simulink model "AGC30Model_ex1_11"  (R2021a)
settings: Solver=ode4  StartTime=stime  StopTime=etime  FixedStep=dtload  RelTol=1e-3
values from neighbouring files (symbols this model uses):
  AL_A = 0.3    [init_lfc_model.m]
  AL_B = 0.3    [init_lfc_model.m]
  DELTA_CC = Delta_cc_ty(TY_CC)    [load_thermal_constants.m]
  DELTA_ST = Delta_st_ty(TY_ST)    [load_thermal_constants.m]
  dtload = 0.1    [initset_dataload.m]
  F0 = 60    [init_inertia_model.m]    (also in initset_inertia.m)
  FFCS0_CC = (WF0_CC-WF_MIN_CC)./(1.0-WF_MIN_CC)    [calc_thermal_init_values.m]    (also in init_thermals.m)
  FGT_CC = Fgt_cc_ty(TY_CC)    [load_thermal_constants.m]
  FX_FB_CC = Fx_fb_cc_ty(:,TY_CC)    [load_thermal_constants.m]
  FX_FB_ST = Fx_fb_st_ty(:,TY_ST)    [load_thermal_constants.m]
  FX_FB_WT = FX_FB_WT_ty(:,TY_WT)    [load_const_hydro_constants.m]
  FX_N_GN_VA = FX_N_GN_VA_ty(:,TY_VA)    [load_var_hydro_constants.m]
  FX_N_PM_VA = FX_N_PM_VA_ty(:,TY_VA)    [load_var_hydro_constants.m]
  FX_PTHD_ST = Fx_pthd_st_ty(:,TY_ST)    [load_thermal_constants.m]
  FX_T_PM_VA = FX_T_PM_VA_ty(:,TY_VA)    [load_var_hydro_constants.m]
  FX_TE1_CC = Fx_te1_cc_ty(:,TY_CC)    [load_thermal_constants.m]
  FX_TE2_CC = Fx_te2_cc_ty(:,TY_CC)    [load_thermal_constants.m]
  FX_Y_GN_VA = FX_Y_GN_VA_ty(:,TY_VA)    [load_var_hydro_constants.m]
  FX_Y_PM_VA = FX_Y_PM_VA_ty(:,TY_VA)    [load_var_hydro_constants.m]
  FY_FB_CC = Fy_fb_cc_ty(:,TY_CC)    [load_thermal_constants.m]
  FY_FB_ST = Fy_fb_st_ty(:,TY_ST)    [load_thermal_constants.m]
  FY_FB_WT = FY_FB_WT_ty(:,TY_WT)    [load_const_hydro_constants.m]
  FY_N_GN_VA = FY_N_GN_VA_ty(:,TY_VA)    [load_var_hydro_constants.m]
  FY_N_PM_VA = FY_N_PM_VA_ty(:,TY_VA)    [load_var_hydro_constants.m]
  FY_PTHD_ST = Fy_pthd_st_ty(:,TY_ST)    [load_thermal_constants.m]
  FY_T_PM_VA = FY_T_PM_VA_ty(:,TY_VA)    [load_var_hydro_constants.m]
  FY_TE1_CC = Fy_te1_cc_ty(:,TY_CC)    [load_thermal_constants.m]
  FY_TE2_CC = Fy_te2_cc_ty(:,TY_CC)    [load_thermal_constants.m]
  FY_Y_GN_VA = FY_Y_GN_VA_ty(:,TY_VA)    [load_var_hydro_constants.m]
  FY_Y_PM_VA = FY_Y_PM_VA_ty(:,TY_VA)    [load_var_hydro_constants.m]
  G_cost = [Cost(:,3) ... (first row only)    [initset_dataload.m]
  G_down_limit = max(G_down_limit, G_out_pre - G_speed*5)    [calc_edc_output.m]    (also in edc.m; initset_dataload.m = csvread('G_down_plan_limit.csv',0,1))
  G_G_ST = G_g_st_ty(TY_ST)    [load_thermal_constants.m]
  G_speed = u(220:249,1)    [calc_edc_output.m]    (also in edc.m; initset_dataload.m = G_speed(:,1))
  GF_CC = [1, 1, 1, 1, 1,            1, 1, 1, 1, 1]    [init_thermal_model.m]
  GF_ST = [1, 1, 1, 1, 1, 1, 1,            1, 1, 1, 1,            1, 1, 1, 1, 1, 1]    [init_thermal_model.m]
  GMW_CC = Gmw_cc_ty(TY_CC)    [load_thermal_constants.m]
  GMW_ST = Gmw_st_ty(TY_ST)    [load_thermal_constants.m]
  GMW_VA = GMW_VA_ty(TY_VA)    [load_var_hydro_constants.m]
  GMW_WT = GMW_WT_ty(TY_WT)    [load_const_hydro_constants.m]
  HC_CC = Hc_cc_ty(TY_CC)    [load_thermal_constants.m]
  HT_CC = Ht_cc_ty(TY_CC)    [load_thermal_constants.m]
  IGV0_CC = WF0_CC    [calc_thermal_init_values.m]    (also in init_thermals.m)
  inertia_input = inertia_input'    [initset_dataload.m]
  K1_CONV_VA = K1_CONV_VA_ty(TY_VA)    [load_var_hydro_constants.m]
  K1_CONV_WT = K1_CONV_WT_ty(TY_WT)    [load_const_hydro_constants.m]
  K2_SERV_VA = K2_SERV_VA_ty(TY_VA)    [load_var_hydro_constants.m]
  K2_SERV_WT = K2_SERV_WT_ty(TY_WT)    [load_const_hydro_constants.m]
  K_A = 0.1    [init_lfc_model.m]
  K_B = 0.1    [init_lfc_model.m]
  K_G_ST = K_g_st_ty(TY_ST)    [load_thermal_constants.m]
  K_IGV_CC = K_igv_cc_ty(TY_CC)    [load_thermal_constants.m]
  K_L = 2.0    (= 2)    [init_inertia_model.m]    (also in initset_inertia.m)
  K_MW_GV_VA = K_MW_GV_VA_ty(TY_VA)    [load_var_hydro_constants.m]
  K_PREF_ST = K_pref_st_ty(TY_ST)    [load_thermal_constants.m]
  K_SD_VA = K_SD_VA_ty(TY_VA)    [load_var_hydro_constants.m]
  K_SD_WT = K_SD_WT_ty(TY_WT)    [load_const_hydro_constants.m]
  K_SEQ_WT = K_SEQ_WT_ty(TY_WT)    [load_const_hydro_constants.m]
  K_TE_CC = K_te_cc_ty(TY_CC)    [load_thermal_constants.m]
  KD_PID_VA = KD_PID_VA_ty(TY_VA)    [load_var_hydro_constants.m]
  KD_PID_WT = KD_PID_WT_ty(TY_WT)    [load_const_hydro_constants.m]
  KD_SG_GN_VA = KD_SG_GN_VA_ty(TY_VA)    [load_var_hydro_constants.m]
  KD_SG_PM_VA = KD_SG_PM_VA_ty(TY_VA)    [load_var_hydro_constants.m]
  KGT_CC = FGT_CC./((TFR_CC-TER_CC)-(TDR_CC-TIR_CC))    [calc_thermal_init_values.m]    (also in init_thermals.m)
  KI_PID_VA = KI_PID_VA_ty(TY_VA)    [load_var_hydro_constants.m]
  KI_PID_WT = KI_PID_WT_ty(TY_WT)    [load_const_hydro_constants.m]
  KI_SG_GN_VA = KI_SG_GN_VA_ty(TY_VA)    [load_var_hydro_constants.m]
  KI_SG_PM_VA = KI_SG_PM_VA_ty(TY_VA)    [load_var_hydro_constants.m]
  KP_A = 1.0    (= 1)    [init_lfc_model.m]
  KP_B = 1.0    (= 1)    [init_lfc_model.m]
  KP_PID_VA = KP_PID_VA_ty(TY_VA)    [load_var_hydro_constants.m]
  KP_PID_WT = KP_PID_WT_ty(TY_WT)    [load_const_hydro_constants.m]
  KP_SG_GN_VA = KP_SG_GN_VA_ty(TY_VA)    [load_var_hydro_constants.m]
  KP_SG_PM_VA = KP_SG_PM_VA_ty(TY_VA)    [load_var_hydro_constants.m]
  KST_CC = (1.0-FGT_CC)./TER_CC    [calc_thermal_init_values.m]    (also in init_thermals.m)
  L_FUEL_CC = L_fuel_cc_ty(TY_CC)    [load_thermal_constants.m]
  L_G_ST = L_g_st_ty(TY_ST)    [load_thermal_constants.m]
  L_IGV_CC = L_igv_cc_ty(TY_CC)    [load_thermal_constants.m]
  L_LL_ST = L_ll_st_ty(TY_ST)    [load_thermal_constants.m]
  L_MWD_CC = L_mwd_cc_ty(TY_CC)    [load_thermal_constants.m]
  L_MWD_GN_VA = L_MWD_GN_VA_ty(TY_VA)    [load_var_hydro_constants.m]
  L_MWD_PM_VA = L_MWD_PM_VA_ty(TY_VA)    [load_var_hydro_constants.m]
  L_MWD_ST = L_mwd_st_ty(TY_ST)    [load_thermal_constants.m]
  L_MWD_WT = L_MWD_WT_ty(TY_WT)    [load_const_hydro_constants.m]
  L_PREF_CC = L_pref_cc_ty(TY_CC)    [load_thermal_constants.m]
  L_PREF_ST = L_pref_st_ty(TY_ST)    [load_thermal_constants.m]
  LFC_cycle = 5.0    (= 5)    [init_lfc_model.m]
  load_input = load_input(:,stime+1:etime+1)    [initset_dataload.m]
  M_VA = M_VA_ty(TY_VA)    [load_var_hydro_constants.m]
  MVABase = 1000    [init_inertia_model.m]    (also in initset_inertia.m)
  MW0_ST = zeros(1,17)    [calc_thermal_init_values.m]    (also in init_thermals.m)
  MW0_WT = zeros(1,2)    [calc_const_hydro_init_values.m]    (also in init_conhydros.m)
  P_G_CONV_WT = P_G_CONV_WT_ty(TY_WT)    [load_const_hydro_constants.m]
  PG_INIT_CC = PMWD_SCHEDULE(1,19:28)'    [calc_thermal_init_values.m]    (also in init_thermals.m)
  PLM_CC = Plm_cc_ty(TY_CC)    [load_thermal_constants.m]
  PLM_ST = Plm_st_ty(TY_ST)    [load_thermal_constants.m]
  PMAX_B = 360.0    (= 360)    [init_lfc_model.m]
  PMIN_B = -360.0    (= -360)    [init_lfc_model.m]
  PMST0_CC = zeros(1, 10)    [calc_thermal_init_values.m]    (also in init_thermals.m)
  PMWD_EDC0 = zeros(1,30)    [init_edc_model.m]    (also in initset_edc.m)
  PMWD_SCHEDULE = u(3:32,1)    [calc_edc_output.m]    (also in edc.m; init_edc_model.m = g_out_input'; initset_edc.m = g_out_input')
  PRC_CC = Prc_cc_ty(TY_CC)    [load_thermal_constants.m]
  PRT_CC = PRC_CC.*(1-EP_CC)    [calc_thermal_init_values.m]    (also in init_thermals.m)
  PTH0_ST = zeros(1,17)    [calc_thermal_init_values.m]    (also in init_thermals.m)
  R_LL_ST = R_ll_st_ty(TY_ST)    [load_thermal_constants.m]
  R_MWD_CC = R_mwd_cc_ty(TY_CC)    [load_thermal_constants.m]
  R_MWD_ST = R_mwd_st_ty(TY_ST)    [load_thermal_constants.m]
  R_PREF_CC = R_pref_cc_ty(TY_CC)    [load_thermal_constants.m]
  RA_A = G_speed'    [init_lfc_model.m]
  RA_B = 96.0    (= 96)    [init_lfc_model.m]
  RATE_GN_VA = RATE_GN_VA_ty(TY_VA)    [load_var_hydro_constants.m]
  RATE_PM_VA = RATE_PM_VA_ty(TY_VA)    [load_var_hydro_constants.m]
  RC_CC = Rc_cc_ty(TY_CC)    [load_thermal_constants.m]
  RT_CC = Rt_cc_ty(TY_CC)    [load_thermal_constants.m]
  SW_T_ST = Sw_t_st_ty(TY_ST)    [load_thermal_constants.m]
  T1_B_ST = T1_b_st_ty(TY_ST)    [load_thermal_constants.m]
  T1_CONV_VA = T1_CONV_VA_ty(TY_VA)    [load_var_hydro_constants.m]
  T1_CONV_WT = T1_CONV_WT_ty(TY_WT)    [load_const_hydro_constants.m]
  T1_G_ST = T1_g_st_ty(TY_ST)    [load_thermal_constants.m]
  T2_B_ST = T2_b_st_ty(TY_ST)    [load_thermal_constants.m]
  ... (+53 more)
undefined symbols (not defined in the file or in its folder): DELTA_B, DiscIntNeverNeededParam, FX_FB_ST_OA, FX_PTHD_ST_OA, FY_FB_ST_OA, FY_PTHD_ST_OA, G_G_ST_OA, K_G_ST_OA, K_PREF_ST_OA, MW0_ST_OA, N_GN_INIT_VA, N_PM_INIT_VA, PLM_B, R_LL_ST_OA, T1_B_ST_OA, T1_G_ST_OA, T2_B_ST_OA, T2_G_ST_OA, T3_B_ST_OA, T4_G_ST_OA, T5_G_ST_OA, T_LL_ST_OA, T_PREF_ST_OA, Y_GN_INIT_VA, Y_PM_INIT_VA
libraries: simulink_extras x87, simulink x42, pid_lib x1
(part 1 of 5)
settings Model: SimulationMode=accelerator  Creator=h-amano  LastModifiedBy=PowerSystemLab
settings SolverCC: AlgebraicLoopSolver=LineSearch
settings DataIOCC: LimitDataPoints=on  SaveFormat=Array  ReturnWorkspaceOutputs=off
settings OptimizationCC: ExpressionDepthLimit=2147483647  LifeSpan=inf
settings DebuggingCC: AlgebraicLoopMsg=none  ArtificialAlgebraicLoopMsg=none  UnderspecifiedInitializationDetection=Classic  MergeDetectMultiDrivingBlocksExec=none  SolverPrmCheckMsg=warning  InheritedTsInSrcMsg=none  MultiTaskRateTransMsg=warning  FcnCallInpInsideContextMsg=warning  StateNameClashWarn=warning  SFUnexpectedBacktrackingDiag=warning  SFNoUnconditionalDefaultTransitionDiag=warning  SFExecutionAtInitializationDiag=none  SFMachineParentedDataDiag=warning  ArithmeticOperatorsInVariantConditions=warning
settings HardwareCC: ProdBitPerPointer=32  ProdBitPerSizeT=32  ProdBitPerPtrDiffT=32  ProdLargestAtomicFloat=None  ProdIntDivRoundTo=Undefined  ProdEndianess=Unspecified  ProdWordSize=32  ProdHWDeviceType=32-bit Generic
settings ModelReferenceCC: PropagateSignalLabelsOutOfModel=off
settings SFSimCC: SimUseLocalCustomCode=off  CustomCodeUndefinedFunction=UseInterfaceOnly
settings RTWCC: RTWUseLocalCustomCode=off
settings CodeAppCC: StateflowObjectComments=on
settings GRTTargetCC: TargetLangStandard=C89/C90 (ANSI)  CombineOutputUpdateFcns=off  GRTInterface=on
settings ConfigComp: CovMetricSettings=dw  CovSaveCumulativeToWorkspaceVar=on  CovSaveSingleToWorkspaceVar=on  CovExternalEMLEnable=off  CovSFcnEnable=off

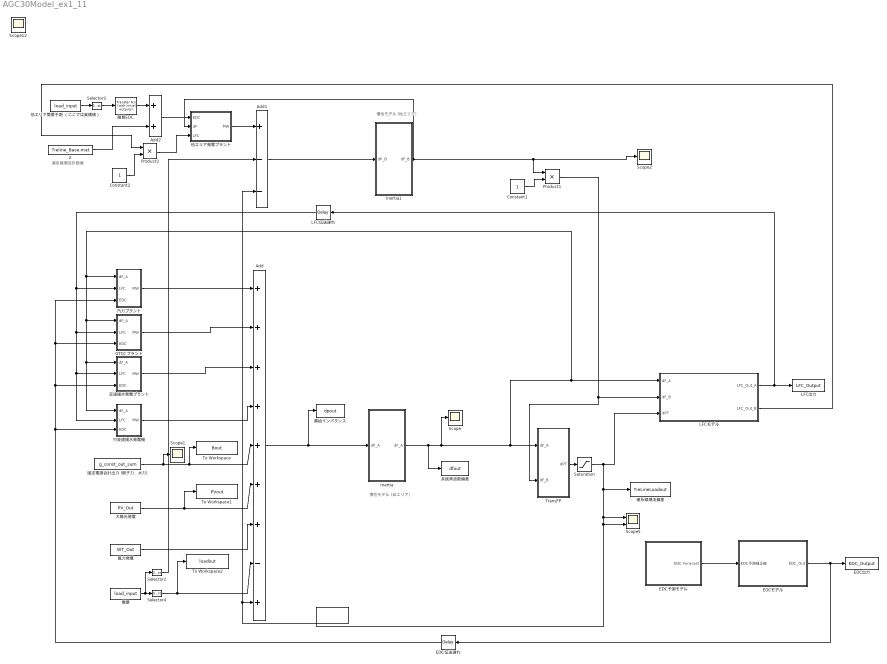
== system AGC30Model_ex1_11 ==
  note: 連系線潮流計画値
  note: 慣性モデル
      | (自エリア)
  note: 慣性モデル
      | (他エリア)
  "  2" : FromFile  FileName=Tieline_Base.mat  SampleTime=dtload
  Add : Sum  Inputs=+++++++-+
  Add1 : Sum  Inputs=+--
  Add2 : Sum
  Constant1 : Constant
  Constant2 : Constant
  EDCモデル : Subsystem
  EDC予測モデル : Subsystem
  EDC伝送遅れ : TransportDelay  DelayTime=3  InitialOutput=PMWD_EDC0
  EDC出力 : ToWorkspace  VariableName=EDC_Output  SampleTime=dtload
      settings: Decimation=10
  GTCCプラント : Subsystem
  Inertia : Subsystem
  Inertia1 : Subsystem
  LFCモデル : Subsystem
  LFC伝送遅れ : TransportDelay  DelayTime=3
  LFC出力 : ToWorkspace  VariableName=LFC_Output  SampleTime=dtload
      settings: Decimation=10
  Product1 : Product
  Product2 : Product
  Saturation : Saturate  UpperLimit=50  LowerLimit=-50
  Scope{,1..2,12} (4 alike) : Scope
  Scope5 : Scope  NumInputPorts=2
  Selector2 : Selector  InputPortWidth=2  IndexOptions=Index vector (dialog)  Indices=[2]  OutputSizes=1
  Selector3 : Selector  InputPortWidth=2  IndexOptions=Index vector (dialog)  Indices=[2]  OutputSizes=1
  Selector4 : Selector  InputPortWidth=2  IndexOptions=Index vector (dialog)  Indices=[1]  OutputSizes=1
  To Workspace : ToWorkspace  VariableName=Bout  SaveFormat=Timeseries  SampleTime=-1
      settings: Decimation=10
  To Workspace1 : ToWorkspace  VariableName=PVout  SaveFormat=Timeseries  SampleTime=-1
      settings: Decimation=10
  To Workspace2 : ToWorkspace  VariableName=loadout  SaveFormat=Timeseries  SampleTime=-1
      settings: Decimation=10
  TransFP : Subsystem
  他エリア発電プラント : Subsystem
  他エリア需要予測 （ここでは実績値） : FromFile  FileName=load_input  SampleTime=dtload
  可変速揚水発電機 : Subsystem
  固定電源合計出力 (原子力，水力) : FromFile  FileName=g_const_out_sum  SampleTime=dtload
  太陽光発電 : FromFile  FileName=PV_Out  SampleTime=dtload
  定速揚水発電プラント : Subsystem
  汽力プラント : Subsystem
  簡易EDC : simulink_extras/Additional Linear/Transfer Fcn (with initial outputs)  N=[1]  D="[200  1]"  Y0=load_input(3,1)  U0=load_input(3,1)
  系統周波数偏差 : ToWorkspace  VariableName=dfout  SampleTime=-1
      settings: Decimation=10  Save2DSignal=2-D array (concatenate along first dimension)
  連系線潮流偏差 : ToWorkspace  VariableName=TieLineLoadout  SampleTime=-1
      settings: Decimation=10  Save2DSignal=2-D array (concatenate along first dimension)
  需給インバランス : ToWorkspace  VariableName=dpout  SampleTime=-1
      settings: Decimation=10  Save2DSignal=2-D array (concatenate along first dimension)
  需要 : FromFile  FileName=load_input  SampleTime=dtload
  風力発電 : FromFile  FileName=WT_Out  SampleTime=dtload
  wires:
  固定電源合計出力 (原子力，水力)/1 -> Scope1/1, To Workspace/1, Add/5
  太陽光発電/1 -> To Workspace1/1, Add/6
  風力発電/1 -> Add/7
  LFCモデル/1(LFC_Out_A) -> LFC出力/1, LFC伝送遅れ/1
  可変速揚水発電機/1(MW) -> Add/4
  定速揚水発電プラント/1(MW) -> Add/3
  汽力プラント/1(MW) -> Add/1
  GTCCプラント/1(MW) -> Add/2
  Add/1 -> 需給インバランス/1, Inertia/1(dP_A)
  Inertia/1(dF_A) -> Scope/1, TransFP/1(dF_A), GTCCプラント/1(dF_A), 可変速揚水発電機/1(dF_A), 定速揚水発電プラント/1(dF_A), 汽力プラント/1(dF_A), LFCモデル/1(dF_A), 系統周波数偏差/1
  Selector4/1 -> To Workspace2/1, Add/8
  EDCモデル/1(EDC_Out) -> EDC出力/1, EDC伝送遅れ/1
  需要/1 -> Selector2/1, Selector4/1
  Selector2/1 -> Add1/2
  他エリア需要予測 （ここでは実績値）/1 -> Selector3/1
  "  2"/1 -> Add2/2
  Selector3/1 -> 簡易EDC/1
  簡易EDC/1 -> Add2/1
  EDC予測モデル/1(EDC Forecast) -> EDCモデル/1(EDC予測補正値)
  EDC伝送遅れ/1 -> 定速揚水発電プラント/3(EDC), GTCCプラント/3(EDC), 汽力プラント/3(EDC), 可変速揚水発電機/3(EDC)
  LFC伝送遅れ/1 -> 汽力プラント/2(LFC), GTCCプラント/2(LFC), 可変速揚水発電機/2(LFC), 定速揚水発電プラント/2(LFC)
  Add2/1 -> 他エリア発電プラント/1(EDC)
  LFCモデル/2(LFC_Out_B) -> Product2/1
  他エリア発電プラント/1(MW) -> Add1/1
  Constant2/1 -> Product2/2
  Product2/1 -> 他エリア発電プラント/3(LFC)
  Inertia1/1(dF_B) -> 他エリア発電プラント/2(dF), Scope2/1, Product1/1
  TransFP/1(dPT) -> Saturation/1
  Add1/1 -> Inertia1/1(dP_B)
  Constant1/1 -> Product1/2
  Product1/1 -> TransFP/2(dF_B), LFCモデル/2(dF_B)
  Saturation/1 -> 連系線潮流偏差/1, Scope5/1, Add/9, Add1/3, Scope5/2, LFCモデル/3(dPT)

== system AGC30Model_ex1_11/EDCモデル ==
  EDC予測補正値 : Inport
  Demux9 : Demux  Outputs=103
      settings: DisplayOption=none
  EDC計算のための入力データ : Subsystem
  Fcn : Fcn  Expr=u-2
  Mux : Mux  Inputs=30
  Mux1 : Mux  Inputs=30
  Mux2 : Mux  Inputs=30
  Mux3 : Mux  Inputs=7
  Mux5 : Mux
  Rate Limiter : RateLimiter  RisingSlewLimit=G_speed/60  FallingSlewLimit=-G_speed/60  SampleTimeMode=inherited  InitialCondition=PMWD_SCHEDULE(1,2:end)
  S-Function1 : S-Function  FunctionName=edc  SFunctionDeploymentMode=off  EnableBusSupport=off
  Switch : Switch  Criteria=u2 ~= 0  Threshold=2
  Switch1 : Switch  Criteria=u2 ~= 0  Threshold=2
  csv_output1 : ToWorkspace  VariableName=PMWD_EDC_O  SampleTime=300
  csv_output10 : ToWorkspace  VariableName=P0_O  SampleTime=300
  csv_output11 : ToWorkspace  VariableName=PMWD_EDC_O1  SampleTime=1
  csv_output2 : ToWorkspace  VariableName=EDC_haibun_O  SampleTime=300
  csv_output3 : ToWorkspace  VariableName=EDC_ERR_O  SampleTime=300
  csv_output4 : ToWorkspace  VariableName=P_OUT_O  SampleTime=300
  csv_output5 : ToWorkspace  VariableName=P_cost_O  SampleTime=300
  csv_output6 : ToWorkspace  VariableName=P_LOAD_A_AD_O  SampleTime=300
  csv_output7 : ToWorkspace  VariableName=P_plan_O  SampleTime=300
  csv_output8 : ToWorkspace  VariableName=G_MODE_O  SampleTime=300
  csv_output9 : ToWorkspace  VariableName=P_CONSTANT_O  SampleTime=300
  hatuden_keikaku : FromWorkspace  VariableName=PMWD_SCHEDULE  SampleTime=-1  ZeroCross=off  OutputAfterFinalValue=Holding final value
  hatudenki_mode : FromWorkspace  VariableName=G_MODE  SampleTime=-1  Interpolate=off  ZeroCross=off  OutputAfterFinalValue=Holding final value
  前回演算時の EDC出力 : UnitDelay  InitialCondition=PMWD_SCHEDULE(1,2:31)  SampleTime=-1  HasFrameUpgradeWarning=on
  発電機の出力変化速度 : Constant  Value=G_speed  SampleTime=-1
  EDC_Out : Outport  VectorParamsAs1DForOutWhenUnconnected=off
  wires:
  Mux/1 -> csv_output1/1, Switch/1
  Demux9/1 -> Mux/1
  Demux9/2 -> Mux/2
  Demux9/3 -> Mux/3
  Demux9/4 -> Mux/4
  Demux9/5 -> Mux/5
  Demux9/6 -> Mux/6
  Demux9/7 -> Mux/7
  Demux9/8 -> Mux/8
  Demux9/9 -> Mux/9
  Demux9/10 -> Mux/10
  Demux9/11 -> Mux/11
  Demux9/12 -> Mux/12
  Demux9/13 -> Mux/13
  Demux9/14 -> Mux/14
  Demux9/15 -> Mux/15
  Demux9/16 -> Mux/16
  Demux9/17 -> Mux/17
  Demux9/18 -> Mux/18
  Demux9/19 -> Mux/19
  Demux9/20 -> Mux/20
  Demux9/21 -> Mux/21
  Demux9/22 -> Mux/22
  Demux9/23 -> Mux/23
  Demux9/24 -> Mux/24
  Demux9/25 -> Mux/25
  Demux9/26 -> Mux/26
  Demux9/27 -> Mux/27
  Demux9/28 -> Mux/28
  Demux9/29 -> Mux/29
  Demux9/30 -> Mux/30
  S-Function1/1 -> Demux9/1
  EDC計算のための入力データ/1(EDC_data) -> Mux5/2
  Mux5/1 -> S-Function1/1
  EDC予測補正値/1 -> Mux5/1
  Mux2/1 -> csv_output8/1
  Demux9/102 -> Mux2/30
  Demux9/101 -> Mux2/29
  Demux9/100 -> Mux2/28
  Demux9/99 -> Mux2/27
  Demux9/98 -> Mux2/26
  Demux9/97 -> Mux2/25
  Demux9/96 -> Mux2/24
  Demux9/95 -> Mux2/23
  Demux9/94 -> Mux2/22
  Demux9/93 -> Mux2/21
  Demux9/92 -> Mux2/20
  Demux9/91 -> Mux2/19
  Demux9/90 -> Mux2/18
  Demux9/89 -> Mux2/17
  Demux9/88 -> Mux2/16
  Demux9/87 -> Mux2/15
  Demux9/85 -> Mux2/13
  Demux9/83 -> Mux2/11
  Demux9/82 -> Mux2/10
  Demux9/81 -> Mux2/9
  Demux9/80 -> Mux2/8
  Demux9/79 -> Mux2/7
  Demux9/78 -> Mux2/6
  Demux9/77 -> Mux2/5
  Demux9/76 -> Mux2/4
  Demux9/75 -> Mux2/3
  Demux9/74 -> Mux2/2
  Demux9/73 -> Mux2/1
  Demux9/72 -> csv_output7/1
  Demux9/71 -> csv_output6/1
  Mux1/1 -> csv_output5/1
  Demux9/41 -> Mux1/1
  Demux9/42 -> Mux1/2
  Demux9/43 -> Mux1/3
  Demux9/44 -> Mux1/4
  Demux9/45 -> Mux1/5
  Demux9/46 -> Mux1/6
  Demux9/47 -> Mux1/7
  Demux9/48 -> Mux1/8
  Demux9/49 -> Mux1/9
  Demux9/50 -> Mux1/10
  Demux9/51 -> Mux1/11
  Demux9/52 -> Mux1/12
  Demux9/53 -> Mux1/13
  Demux9/54 -> Mux1/14
  Demux9/55 -> Mux1/15
  Demux9/56 -> Mux1/16
  Demux9/57 -> Mux1/17
  Demux9/58 -> Mux1/18
  Demux9/59 -> Mux1/19
  Demux9/61 -> Mux1/21
  Demux9/62 -> Mux1/22
  Demux9/63 -> Mux1/23
  Demux9/64 -> Mux1/24
  Demux9/65 -> Mux1/25
  Demux9/66 -> Mux1/26
  Demux9/67 -> Mux1/27
  Demux9/68 -> Mux1/28
  Demux9/69 -> Mux1/29
  Demux9/70 -> Mux1/30
  Demux9/31 -> Mux3/1
  Demux9/32 -> Mux3/2
  Demux9/33 -> Mux3/3
  Demux9/34 -> Mux3/4
  Demux9/35 -> Mux3/5
  Demux9/36 -> Mux3/6
  Demux9/37 -> Mux3/7
  Mux3/1 -> csv_output9/1
  Demux9/60 -> Mux1/20
  Demux9/38 -> csv_output2/1
  Demux9/39 -> csv_output3/1
  Demux9/40 -> csv_output4/1
  Demux9/84 -> Mux2/12
  Demux9/86 -> Mux2/14
  Demux9/103 -> csv_output10/1
  hatudenki_mode/1 -> Fcn/1, Switch/2
  hatuden_keikaku/1 -> Switch1/3, Switch/3
  Switch/1 -> Switch1/1
  Fcn/1 -> Switch1/2
  前回演算時の EDC出力/1 -> Mux5/4
  発電機の出力変化速度/1 -> Mux5/3
  Switch1/1 -> Rate Limiter/1, 前回演算時の EDC出力/1, EDC_Out/1
  Rate Limiter/1 -> csv_output11/1

== system AGC30Model_ex1_11/EDC予測モデル ==
  EDC予測データ : ToWorkspace  VariableName=load_forcast_out  SampleTime=-1
      settings: Decimation=10  Save2DSignal=2-D array (concatenate along first dimension)
  Gain : Gain  Gain=1/200
  Integrator : Integrator  InitialConditionSource=external
  Mux : Mux  Inputs=2
  Mux1 : Mux  Inputs=3
  Scope : Scope
  Scope1 : Scope
  Selector2 : Selector  InputPortWidth=2  IndexOptions=Index vector (dialog)  Indices=[1]  OutputSizes=1
  Subtract : Sum  Inputs=+--
  Sum : Sum  Inputs=|+-
  Sum1 : Sum  Inputs=++|
  Sum2 : Sum  Inputs=|+-
  太陽光発電 : FromFile  FileName=PV_Out  SampleTime=dtload
  発電計画時の予測需要 : FromFile  FileName=load_forecast_input  SampleTime=dtload
  発電計画時の予測需要 （5分先） : FromFile  FileName=load_forecast_300s_input  SampleTime=dtload
  需要 : FromFile  FileName=load_input  SampleTime=dtload
  風力発電 : FromFile  FileName=WT_Out  SampleTime=dtload
  EDC Forecast : Outport  VectorParamsAs1DForOutWhenUnconnected=off
  wires:
  Gain/1 -> Integrator/1
  Sum1/1 -> Mux1/3, EDC Forecast/1
  需要/1 -> Selector2/1
  発電計画時の予測需要/1 -> Mux1/2, Sum/2, Mux/1
  Subtract/1 -> Mux1/1, Sum/1
  Mux/1 -> Scope/1
  Sum/1 -> Integrator/2, Sum2/1
  Sum2/1 -> Gain/1
  発電計画時の予測需要 （5分先）/1 -> Mux/2, Sum1/2
  Integrator/1 -> Sum1/1, Sum2/2
  Mux1/1 -> Scope1/1, EDC予測データ/1
  Selector2/1 -> Subtract/1
  太陽光発電/1 -> Subtract/2
  風力発電/1 -> Subtract/3

== system AGC30Model_ex1_11/GTCCプラント ==
  dF_A : Inport
  LFC : Inport  Port=2
  EDC : Inport  Port=3
  Add : Sum  Inputs=+
  EDC_Gtcc1 : Selector  InputPortWidth=AGCNum_E  IndexOptions=Index vector (dialog)  Indices=[18]  OutputSizes=1
  GTCC1 : Subsystem
  GTCCプラント出力 : ToWorkspace  VariableName=Combine_Output  SampleTime=-1
      settings: Decimation=10  Save2DSignal=2-D array (concatenate along first dimension)
  LFC_Gtcc1 : Selector  InputPortWidth=AGCNum_L  IndexOptions=Index vector (dialog)  Indices=[18]  OutputSizes=1
  Mux : Mux  Inputs=1
  To Workspace : ToWorkspace  VariableName=GTCC  SaveFormat=Timeseries  SampleTime=-1
      settings: Decimation=10
  MW : Outport  VectorParamsAs1DForOutWhenUnconnected=off
  wires:
  GTCC1/1(タービン出力(MW)) -> Add/1, To Workspace/1, Mux/1
  LFC/1 -> LFC_Gtcc1/1
  dF_A/1 -> GTCC1/3(周波数偏差(Hz))
  Mux/1 -> GTCCプラント出力/1
  LFC_Gtcc1/1 -> GTCC1/2(LFC指令値(MW))
  Add/1 -> MW/1
  EDC_Gtcc1/1 -> GTCC1/1(EDC指令値(MW))
  EDC/1 -> EDC_Gtcc1/1

== system AGC30Model_ex1_11/Inertia ==
  note: 系統容量
  note: 慣性定数
  note: 需給インバランス
      | (ΔP)
  dP_A : Inport  SampleTime=0.1
  "  1" : FromFile  FileName=inertia_input.mat  SampleTime=dtload
  "  2" : FromFile  FileName=load_input.mat  SampleTime=dtload
  Add2 : Sum  Inputs=+-
  Divide : Product  Inputs=/*
  Divide1 : Product  Inputs=/*
  Divide2 : Product  Inputs=**
  Selector1 : Selector  InputPortWidth=2  IndexOptions=Index vector (dialog)  Indices=[1]  OutputSizes=1
  Selector2 : Selector  InputPortWidth=2  IndexOptions=Index vector (dialog)  Indices=[1]  OutputSizes=1
  Transfer Fcn : TransferFcn  Denominator=[1 0]
  基準周波数 : Gain  Gain=F0
  系統容量基準値 : Constant  Value=MVABase
  負荷周波数特性係数 : Gain  Gain=K_L
  dF_A : Outport  VectorParamsAs1DForOutWhenUnconnected=off
  wires:
  負荷周波数特性係数/1 -> Divide2/2
  Divide/1 -> Divide1/2
  dP_A/1 -> Add2/1
  "  1"/1 -> Selector2/1
  Selector1/1 -> Divide2/1  "P_LOAD_A"
  基準周波数/1 -> dF_A/1  "d_F_A"
  Divide1/1 -> Transfer Fcn/1
  "  2"/1 -> Selector1/1
  Transfer Fcn/1 -> 負荷周波数特性係数/1, 基準周波数/1
  Add2/1 -> Divide/2
  Divide2/1 -> Add2/2
  系統容量基準値/1 -> Divide/1
  Selector2/1 -> Divide1/1  "M_0_A"

== system AGC30Model_ex1_11/Inertia1 ==
  note: 系統容量
  note: 慣性定数
  note: 需給インバランス
      | (ΔP)
  dP_B : Inport  SampleTime=0.1
  "  1" : FromFile  FileName=inertia_input.mat  SampleTime=dtload
  "  2" : FromFile  FileName=load_input.mat  SampleTime=dtload
  Add1 : Sum  Inputs=+-
  Divide : Product  Inputs=/*
  Divide1 : Product  Inputs=/*
  Divide2 : Product  Inputs=**
  Selector1 : Selector  InputPortWidth=2  IndexOptions=Index vector (dialog)  Indices=[2]  OutputSizes=1
  Selector2 : Selector  InputPortWidth=2  IndexOptions=Index vector (dialog)  Indices=[2]  OutputSizes=1
  Transfer Fcn : TransferFcn  Denominator=[1 0]
  基準周波数 : Gain  Gain=F0
  系統容量基準値 : Constant  Value=MVABase
  負荷周波数特性係数 : Gain  Gain=K_L
  dF_B : Outport  VectorParamsAs1DForOutWhenUnconnected=off
  wires:
  Transfer Fcn/1 -> 基準周波数/1, 負荷周波数特性係数/1
  "  2"/1 -> Selector1/1
  Divide1/1 -> Transfer Fcn/1
  基準周波数/1 -> dF_B/1  "d_F_B"
  "  1"/1 -> Selector2/1
  dP_B/1 -> Add1/1
  Selector2/1 -> Divide1/1  "M_0_A"
  系統容量基準値/1 -> Divide/1
  負荷周波数特性係数/1 -> Divide2/2
  Selector1/1 -> Divide2/1  "P_LOAD_A"
  Divide2/1 -> Add1/2
  Add1/1 -> Divide/2
  Divide/1 -> Divide1/2

== system AGC30Model_ex1_11/LFCモデル ==
  note: 連系線潮流計画値
  note: 系統容量
      | (需要データ)
  dF_A : Inport  SampleTime=dtload
  dF_B : Inport  Port=2  SampleTime=dtload
  dPT : Inport  Port=3  SampleTime=dtload
  "  1" : FromFile  FileName=load_input.mat  SampleTime=dtload
  "  2" : FromFile  FileName=Tieline_Base.mat  SampleTime=dtload
  Rate Transition : RateTransition  Deterministic=off  InitialCondition=load_input([2,3],1)  OutPortSampleTime=LFC_cycle
  Rate Transition1 : RateTransition  Deterministic=off  OutPortSampleTime=LFC_cycle
  Sum : Sum  Inputs=-+
  TBC/FFC 切替Switch : ManualSwitch
  TBC/FFC 切替Switch : ManualSwitch
  他エリア FFC方式 : Subsystem
  他エリア TBC方式 : Subsystem
  自エリア TBC方式 : Subsystem
  自エリアFFC方式 : Subsystem
  LFC_Out_A : Outport  VectorParamsAs1DForOutWhenUnconnected=off
  LFC_Out_B : Outport  Port=2  VectorParamsAs1DForOutWhenUnconnected=off
  wires:
  "  1"/1 -> Rate Transition/1
  Rate Transition/1 -> 自エリア TBC方式/1(系統容量(MW)), 自エリアFFC方式/1(系統容量(MW)), 他エリア TBC方式/1(系統容量(MW)), 他エリア FFC方式/1(系統容量(MW))
  自エリア TBC方式/1(LFC指令値(MW)) -> TBC/FFC 切替Switch/1
  自エリアFFC方式/1(LFC指令値(MW)) -> TBC/FFC 切替Switch/2
  TBC/FFC 切替Switch/1 -> LFC_Out_A/1
  dF_A/1 -> 自エリア TBC方式/2(周波数偏差(Hz)), 自エリアFFC方式/2(周波数偏差(Hz))
  他エリア TBC方式/1(LFC指令値(MW)) -> TBC/FFC 切替Switch/1
  他エリア FFC方式/1(LFC指令値(MW)) -> TBC/FFC 切替Switch/2
  TBC/FFC 切替Switch/1 -> LFC_Out_B/1
  dF_B/1 -> 他エリア TBC方式/2(周波数偏差(Hz)), 他エリア FFC方式/2(周波数偏差(Hz))
  "  2"/1 -> Sum/1
  dPT/1 -> Sum/2
  Sum/1 -> Rate Transition1/1
  Rate Transition1/1 -> 自エリア TBC方式/3(連系線潮流偏差(MW)), 他エリア TBC方式/3(連系線潮流偏差(Hz))

== system AGC30Model_ex1_11/TransFP ==
  dF_A : Inport
  dF_B : Inport  Port=2
  "  2" : FromFile  FileName=inertia_input.mat  SampleTime=dtload
  Add1 : Sum  Inputs=-+
  Add2 : Sum
  Constant1 : Constant  Value=2*pi/(F0*T_0^2)  SampleTime=dtload
  Divide : Product  Inputs=**
  Divide1 : Product  Inputs=//
  Divide2 : Product  Inputs=//
  Divide3 : Product  Inputs=/*
  F_0 : Gain  Gain=2*pi
  F_1 : Gain  Gain=2*pi
  Integrator : Integrator  InitialCondition=Tieline_Base(2,1)/(2*pi/(F0*T_0^2))*(1/(MVABase*inertia_input(2,1))+1/(MVABase*inertia_input(3,1)))
  Selector1 : Selector  InputPortWidth=2  IndexOptions=Index vector (dialog)  Indices=[1]  OutputSizes=1
  Selector3 : Selector  InputPortWidth=2  IndexOptions=Index vector (dialog)  Indices=[2]  OutputSizes=1
  系統容量基準値 : Constant  Value=MVABase
  dPT : Outport  SampleTime=dtload  VectorParamsAs1DForOutWhenUnconnected=off
  wires:
  Selector3/1 -> Divide2/1  "M_0_B"
  Selector1/1 -> Divide1/1  "M_0_A"
  Add1/1 -> Integrator/1
  "  2"/1 -> Selector3/1, Selector1/1
  dF_A/1 -> F_0/1
  dF_B/1 -> F_1/1
  Add2/1 -> Divide3/1
  Divide1/1 -> Add2/1
  Divide2/1 -> Add2/2
  Constant1/1 -> Divide3/2
  Divide3/1 -> Divide/1  "T_AB"
  F_0/1 -> Add1/1
  Divide/1 -> dPT/1  "DPT"
  F_1/1 -> Add1/2
  Integrator/1 -> Divide/2
  系統容量基準値/1 -> Divide2/2, Divide1/2

== system AGC30Model_ex1_11/他エリア発電プラント ==
  EDC : Inport
  dF : Inport  Port=2
  LFC : Inport  Port=3
  Scope : Scope  NumInputPorts=4
  他エリアモデル : Subsystem
  MW : Outport  VectorParamsAs1DForOutWhenUnconnected=off
  wires:
  他エリアモデル/1(タービン出力(MW)) -> Scope/4, MW/1
  EDC/1 -> Scope/3, 他エリアモデル/1(EDC指令値(MW))
  LFC/1 -> Scope/2, 他エリアモデル/2(LFC指令値(MW))
  dF/1 -> Scope/1, 他エリアモデル/3(周波数偏差(Hz))

== system AGC30Model_ex1_11/可変速揚水発電機 ==
  dF_A : Inport
  LFC : Inport  Port=2
  EDC : Inport  Port=3
  可変速揚水 : Subsystem
  可変速揚水機出力 : ToWorkspace  VariableName=C_Water_Output  SampleTime=-1
      settings: Decimation=10  Save2DSignal=2-D array (concatenate along first dimension)
  MW : Outport  VectorParamsAs1DForOutWhenUnconnected=off
  wires:
  EDC/1 -> 可変速揚水/1(EDC指令値 (MW))
  LFC/1 -> 可変速揚水/2(LFC指令値 (MW))
  dF_A/1 -> 可変速揚水/3(周波数偏差 (Hz))
  可変速揚水/1(発電機出力・揚水入力 (MW)) -> 可変速揚水機出力/1, MW/1

== system AGC30Model_ex1_11/定速揚水発電プラント ==
  dF_A : Inport
  LFC : Inport  Port=2
  EDC : Inport  Port=3
  Add : Sum
  EDC_Wt1 : Selector  InputPortWidth=AGCNum_E  IndexOptions=Index vector (dialog)  Indices=[28]  OutputSizes=1
  EDC_Wt2 : Selector  InputPortWidth=AGCNum_E  IndexOptions=Index vector (dialog)  Indices=[29]  OutputSizes=1
  LFC_Wt1 : Selector  InputPortWidth=AGCNum_L  IndexOptions=Index vector (dialog)  Indices=[28]  OutputSizes=1
  LFC_Wt2 : Selector  InputPortWidth=AGCNum_L  IndexOptions=Index vector (dialog)  Indices=[29]  OutputSizes=1
  Water1 : Subsystem
  Water2 : Subsystem
  定速揚水プラント出力1 : ToWorkspace  VariableName=Water_Output1  SampleTime=-1
      settings: Decimation=10  Save2DSignal=2-D array (concatenate along first dimension)
  定速揚水プラント出力2 : ToWorkspace  VariableName=Water_Output2  SampleTime=-1
      settings: Decimation=10  Save2DSignal=2-D array (concatenate along first dimension)
  MW : Outport  VectorParamsAs1DForOutWhenUnconnected=off
  wires:
  EDC/1 -> EDC_Wt2/1, EDC_Wt1/1
  LFC/1 -> LFC_Wt1/1, LFC_Wt2/1
  dF_A/1 -> Water1/3(周波数偏差(Hz)1), Water2/3(周波数偏差(Hz)1)
  Water1/1(タービン出力(MW)) -> 定速揚水プラント出力1/1, Add/1
  Water2/1(タービン出力(MW)) -> 定速揚水プラント出力2/1, Add/2
  Add/1 -> MW/1
  EDC_Wt1/1 -> Water1/1(EDC指令値(MW))
  LFC_Wt1/1 -> Water1/2(LFC指令値(MW)1)
  LFC_Wt2/1 -> Water2/2(LFC指令値(MW)1)
  EDC_Wt2/1 -> Water2/1(EDC指令値(MW))

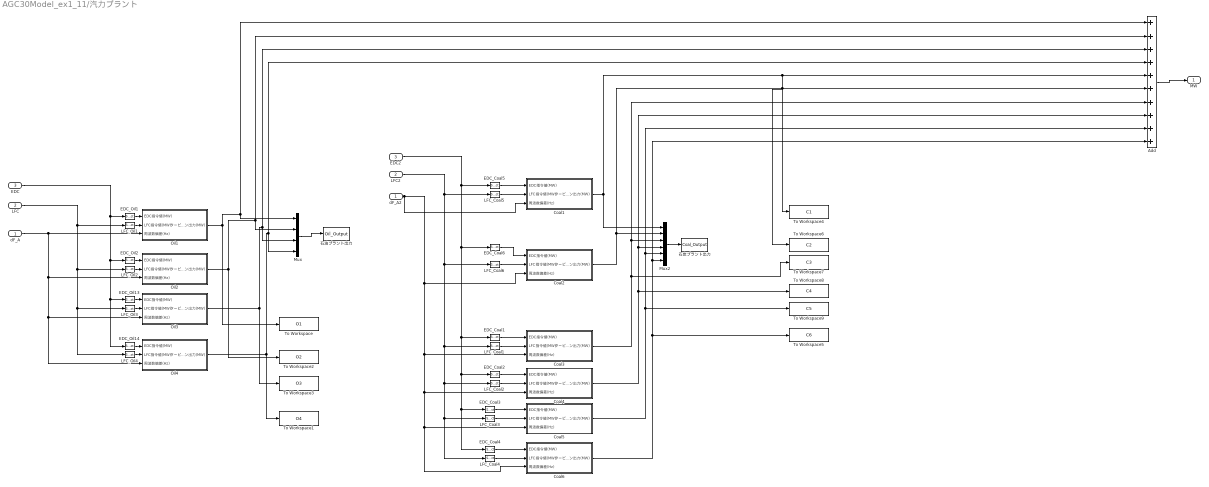
== system AGC30Model_ex1_11/汽力プラント ==
  dF_A : Inport
  LFC : Inport  Port=2
  EDC : Inport  Port=3
  Add : Sum  Inputs=++++++++++
  Coal1 : Subsystem
  Coal2 : Subsystem
  Coal3 : Subsystem
  Coal4 : Subsystem
  Coal5 : Subsystem
  Coal6 : Subsystem
  EDC2 : InportShadow  Port=3
  EDC_Coal1 : Selector  InputPortWidth=AGCNum_E  IndexOptions=Index vector (dialog)  Indices=[8]  OutputSizes=1
  EDC_Coal2 : Selector  InputPortWidth=AGCNum_E  IndexOptions=Index vector (dialog)  Indices=[9]  OutputSizes=1
  EDC_Coal3 : Selector  InputPortWidth=AGCNum_E  IndexOptions=Index vector (dialog)  Indices=[10]  OutputSizes=1
  EDC_Coal4 : Selector  InputPortWidth=AGCNum_E  IndexOptions=Index vector (dialog)  Indices=[11]  OutputSizes=1
  EDC_Coal5 : Selector  InputPortWidth=AGCNum_E  IndexOptions=Index vector (dialog)  Indices=[6]  OutputSizes=1
  EDC_Coal6 : Selector  InputPortWidth=AGCNum_E  IndexOptions=Index vector (dialog)  Indices=[7]  OutputSizes=1
  EDC_Oil1 : Selector  InputPortWidth=AGCNum_E  IndexOptions=Index vector (dialog)  Indices=[1]  OutputSizes=1
  EDC_Oil13 : Selector  InputPortWidth=AGCNum_E  IndexOptions=Index vector (dialog)  Indices=[3]  OutputSizes=1
  EDC_Oil14 : Selector  InputPortWidth=AGCNum_E  IndexOptions=Index vector (dialog)  Indices=[4]  OutputSizes=1
  EDC_Oil2 : Selector  InputPortWidth=AGCNum_E  IndexOptions=Index vector (dialog)  Indices=[2]  OutputSizes=1
  LFC2 : InportShadow  Port=2
  LFC_Coal1 : Selector  InputPortWidth=AGCNum_L  IndexOptions=Index vector (dialog)  Indices=[8]  OutputSizes=1
  LFC_Coal2 : Selector  InputPortWidth=AGCNum_L  IndexOptions=Index vector (dialog)  Indices=[9]  OutputSizes=1
  LFC_Coal3 : Selector  InputPortWidth=AGCNum_L  IndexOptions=Index vector (dialog)  Indices=[10]  OutputSizes=1
  LFC_Coal4 : Selector  InputPortWidth=AGCNum_L  IndexOptions=Index vector (dialog)  Indices=[11]  OutputSizes=1
  LFC_Coal5 : Selector  InputPortWidth=AGCNum_L  IndexOptions=Index vector (dialog)  Indices=[6]  OutputSizes=1
  LFC_Coal6 : Selector  InputPortWidth=AGCNum_L  IndexOptions=Index vector (dialog)  Indices=[7]  OutputSizes=1
  LFC_Oil1 : Selector  InputPortWidth=AGCNum_L  IndexOptions=Index vector (dialog)  Indices=[1]  OutputSizes=1
  LFC_Oil2 : Selector  InputPortWidth=AGCNum_L  IndexOptions=Index vector (dialog)  Indices=[2]  OutputSizes=1
  LFC_Oil3 : Selector  InputPortWidth=AGCNum_L  IndexOptions=Index vector (dialog)  Indices=[3]  OutputSizes=1
  LFC_Oil4 : Selector  InputPortWidth=AGCNum_L  IndexOptions=Index vector (dialog)  Indices=[4]  OutputSizes=1
  Mux : Mux
  Mux2 : Mux  Inputs=6
  Oil1 : Subsystem
  Oil2 : Subsystem
  Oil3 : Subsystem
  Oil4 : Subsystem
  To Workspace : ToWorkspace  VariableName=O1  SaveFormat=Timeseries  SampleTime=-1
      settings: Decimation=10
  To Workspace1 : ToWorkspace  VariableName=O4  SaveFormat=Timeseries  SampleTime=-1
      settings: Decimation=10
  To Workspace2 : ToWorkspace  VariableName=O2  SaveFormat=Timeseries  SampleTime=-1
      settings: Decimation=10
  To Workspace3 : ToWorkspace  VariableName=O3  SaveFormat=Timeseries  SampleTime=-1
      settings: Decimation=10
  To Workspace4 : ToWorkspace  VariableName=C1  SaveFormat=Timeseries  SampleTime=-1
      settings: Decimation=10
  To Workspace5 : ToWorkspace  VariableName=C6  SaveFormat=Timeseries  SampleTime=-1
      settings: Decimation=10
  To Workspace6 : ToWorkspace  VariableName=C2  SaveFormat=Timeseries  SampleTime=-1
      settings: Decimation=10
  To Workspace7 : ToWorkspace  VariableName=C3  SaveFormat=Timeseries  SampleTime=-1
      settings: Decimation=10
  To Workspace8 : ToWorkspace  VariableName=C4  SaveFormat=Timeseries  SampleTime=-1
      settings: Decimation=10
  To Workspace9 : ToWorkspace  VariableName=C5  SaveFormat=Timeseries  SampleTime=-1
      settings: Decimation=10
  dF_A2 : InportShadow
  石油プラント出力 : ToWorkspace  VariableName=Oil_Output  SampleTime=-1
      settings: Decimation=10  Save2DSignal=2-D array (concatenate along first dimension)
  石炭プラント出力 : ToWorkspace  VariableName=Coal_Output  SampleTime=-1
      settings: Decimation=10  Save2DSignal=2-D array (concatenate along first dimension)
  MW : Outport  VectorParamsAs1DForOutWhenUnconnected=off
  wires:
  LFC/1 -> LFC_Oil1/1, LFC_Oil3/1, LFC_Oil4/1, LFC_Oil2/1
  dF_A/1 -> Oil2/3(周波数偏差(Hz)), Oil3/3(周波数偏差(Hz)), Oil4/3(周波数偏差(Hz)), Oil1/3(周波数偏差(Hz))
  Mux/1 -> 石油プラント出力/1
  Oil1/1(タービン出力(MW)) -> To Workspace/1, Add/1, Mux/1
  Oil2/1(タービン出力(MW)) -> To Workspace2/1, Add/2, Mux/2
  Oil3/1(タービン出力(MW)) -> To Workspace3/1, Add/3, Mux/3
  Oil4/1(タービン出力(MW)) -> To Workspace1/1, Add/4, Mux/4
  Mux2/1 -> 石炭プラント出力/1
  Coal3/1(タービン出力(MW)) -> Add/7, Mux2/3, To Workspace7/1
  Coal5/1(タービン出力(MW)) -> To Workspace9/1, Mux2/5, Add/9
  Coal6/1(タービン出力(MW)) -> To Workspace5/1, Mux2/6, Add/10
  LFC_Oil1/1 -> Oil1/2(LFC指令値(MW))
  LFC_Oil2/1 -> Oil2/2(LFC指令値(MW))
  LFC_Oil4/1 -> Oil4/2(LFC指令値(MW))
  LFC_Coal1/1 -> Coal3/2(LFC指令値(MW))
  LFC_Coal2/1 -> Coal4/2(LFC指令値(MW))
  LFC_Coal3/1 -> Coal5/2(LFC指令値(MW))
  LFC_Coal4/1 -> Coal6/2(LFC指令値(MW))
  Add/1 -> MW/1
  Coal4/1(タービン出力(MW)) -> To Workspace8/1, Mux2/4, Add/8
  EDC_Oil1/1 -> Oil1/1(EDC指令値(MW))
  EDC_Oil2/1 -> Oil2/1(EDC指令値(MW))
  EDC_Oil14/1 -> Oil4/1(EDC指令値(MW))
  EDC_Coal3/1 -> Coal5/1(EDC指令値(MW))
  EDC_Coal2/1 -> Coal4/1(EDC指令値(MW))
  EDC_Coal1/1 -> Coal3/1(EDC指令値(MW))
  EDC_Coal4/1 -> Coal6/1(EDC指令値(MW))
  EDC_Oil13/1 -> Oil3/1(EDC指令値(MW))
  LFC_Oil3/1 -> Oil3/2(LFC指令値(MW))
  EDC/1 -> EDC_Oil1/1, EDC_Oil2/1, EDC_Oil13/1, EDC_Oil14/1
  LFC_Coal5/1 -> Coal1/2(LFC指令値(MW))
  EDC_Coal5/1 -> Coal1/1(EDC指令値(MW))
  LFC2/1 -> LFC_Coal5/1, LFC_Coal6/1, LFC_Coal2/1, LFC_Coal3/1, LFC_Coal4/1, LFC_Coal1/1
  EDC2/1 -> EDC_Coal5/1, EDC_Coal1/1, EDC_Coal4/1, EDC_Coal3/1, EDC_Coal2/1, EDC_Coal6/1
  dF_A2/1 -> Coal1/3(周波数偏差(Hz)), Coal2/3(周波数偏差(Hz)), Coal5/3(周波数偏差(Hz)), Coal6/3(周波数偏差(Hz)), Coal4/3(周波数偏差(Hz)), Coal3/3(周波数偏差(Hz))
  EDC_Coal6/1 -> Coal2/1(EDC指令値(MW))
  LFC_Coal6/1 -> Coal2/2(LFC指令値(MW))
  Coal1/1(タービン出力(MW)) -> Mux2/1, To Workspace4/1, Add/5
  Coal2/1(タービン出力(MW)) -> Mux2/2, To Workspace6/1, Add/6

== system AGC30Model_ex1_11/EDCモデル/EDC計算のための入力データ ==
  note: メモ（電中研）：出力上限は
      | 停止を考慮した時系列データ
      | を設定（停止に先立って上限
      | を絞る）
  MinMax : MinMax  Inputs=2
  Mux6 : Mux  Inputs=7
  hatuden_keikaku : FromWorkspace  VariableName=PMWD_SCHEDULE  SampleTime=-1  ZeroCross=off  OutputAfterFinalValue=Holding final value
  hatuden_keikaku1 : FromWorkspace  VariableName=P_CONSTANT  SampleTime=-1  ZeroCross=off  OutputAfterFinalValue=Holding final value
  hatudenki_kagen : Constant  Value=G_down_limit  SampleTime=-1
  hatudenki_mode : FromWorkspace  VariableName=G_MODE  SampleTime=-1  ZeroCross=off  OutputAfterFinalValue=Holding final value
  hatudenki_mode1 : FromWorkspace  VariableName=G_up_limit2  SampleTime=-1  Interpolate=off  ZeroCross=off  OutputAfterFinalValue=Holding final value
  nenryouhi : Constant  Value=G_cost  SampleTime=-1
  renkeisen : FromWorkspace  VariableName=P0  SampleTime=-1  ZeroCross=off  OutputAfterFinalValue=Holding final value
  EDC_data : Outport  VectorParamsAs1DForOutWhenUnconnected=off
  wires:
  Mux6/1 -> EDC_data/1
  hatuden_keikaku/1 -> Mux6/2
  nenryouhi/1 -> Mux6/5
  hatudenki_mode/1 -> Mux6/4
  hatuden_keikaku1/1 -> Mux6/3
  renkeisen/1 -> Mux6/1
  hatudenki_mode1/1 -> Mux6/6, MinMax/1
  hatudenki_kagen/1 -> MinMax/2
  MinMax/1 -> Mux6/7

== system AGC30Model_ex1_11/GTCCプラント/GTCC1 ==
  EDC指令値(MW) : Inport
  LFC指令値(MW) : Inport  Port=2
  周波数偏差(Hz) : Inport  Port=3
  FFCS : Scope
  Hz->pu : Gain  Gain=1/F0
  IGV : Scope
  IGV制御 : Subsystem
  MW->pu : Gain  Gain=1/GMW_CC(1)
  MWD(MW) : Sum
  Mux : Mux  Inputs=3
  Mux1 : Mux  Inputs=2
  Pm : Scope
  Pmgt : Scope
  Pmst : Scope
  Te : Scope
  W : Scope
  Wf : Scope
  pu->MW : Gain  Gain=GMW_CC(1)
  ガスタービン : Subsystem
  出力切替不連続防止 : Subsystem
  排ガス温度制御 : Subsystem
  燃料制御 : Subsystem
  蒸気タービン : Subsystem
  負荷制限制御 : Subsystem
  軸出力 : Sum
  速度・負荷制御 : Subsystem
  運転モード : simulink/Logic and Bit Operations/Compare To Constant  relop=>=  const=L_MWD_CC(1)*GMW_CC(1)  OutDataTypeStr=boolean
  タービン出力(MW) : Outport  VectorParamsAs1DForOutWhenUnconnected=off
  wires:
  ガスタービン/1(ガスタービン出力) -> IGV制御/2(ガスタービン出力), 排ガス温度制御/3(ガスタービン出力), 軸出力/1, Pmgt/1
  速度・負荷制御/1(速度・負荷制御信号) -> Mux/1, 燃料制御/1(速度・負荷制御信号), 負荷制限制御/1(速度・負荷制御信号)
  ガスタービン/3(排ガス温度) -> Te/1, 排ガス温度制御/2(排ガス温度), 蒸気タービン/2(排ガス温度)
  燃料制御/1(燃料流量) -> Wf/1, ガスタービン/1(燃料流量)
  Hz->pu/1 -> ガスタービン/2(周波数偏差), 燃料制御/4(周波数偏差), 負荷制限制御/3(周波数偏差), 速度・負荷制御/3(周波数偏差)
  IGV制御/1(IGV開度) -> IGV/1, ガスタービン/3(IGV開度)
  蒸気タービン/1(蒸気タービン出力) -> Pmst/1, 軸出力/2
  排ガス温度制御/2(排ガス温度計測値) -> IGV制御/1(排ガス温度計測値)
  負荷制限制御/1(負荷制限制御信号) -> Mux/2, 燃料制御/2(負荷制限制御信号)
  排ガス温度制御/1(排ガス温度制御信号) -> Mux/3, 燃料制御/3(排ガス温度制御信号), 速度・負荷制御/5(排ガス温度制御信号)
  MWD(MW)/1 -> MW->pu/1
  軸出力/1 -> 速度・負荷制御/1(軸出力), 出力切替不連続防止/1(モデル)
  MW->pu/1 -> 出力切替不連続防止/3(出力指令値), Mux1/2, 速度・負荷制御/2(出力指令値)
  LFC指令値(MW)/1 -> MWD(MW)/2
  周波数偏差(Hz)/1 -> Hz->pu/1
  出力切替不連続防止/1(出力) -> Mux1/1, pu->MW/1
  EDC指令値(MW)/1 -> 運転モード/1, MWD(MW)/1
  pu->MW/1 -> タービン出力(MW)/1
  運転モード/1 -> 出力切替不連続防止/2(運転モード)
  Mux1/1 -> Pm/1
  ガスタービン/2("空気流量 ") -> W/1, 蒸気タービン/1(空気流量)
  燃料制御/2(燃料制御信号) -> 速度・負荷制御/4(燃料流量制御信号), 負荷制限制御/2(燃料流量制御信号), 排ガス温度制御/1(燃料流量制御信号)
  Mux/1 -> FFCS/1

== system AGC30Model_ex1_11/LFCモデル/他エリア FFC方式 ==
  系統容量(MW) : Inport
  周波数偏差(Hz) : Inport  Port=2
  Constant10 : Constant  Value=XF_B  SampleTime=LFC_cycle
  Constant12 : Constant  Value=XAR_B  SampleTime=LFC_cycle
  Discrete-Time Integrator : DiscreteIntegrator  gainval=KI_B  SampleTime=LFC_cycle  ICPrevOutput=DiscIntNeverNeededParam  ICPrevScaledInput=DiscIntNeverNeededParam
  Embedded MATLAB Function4 : MATLAB Function  TreatAsAtomicUnit=on
  Embedded MATLAB Function5 : MATLAB Function  TreatAsAtomicUnit=on
  Gain1 : Gain  Gain=KP_B  SampleTime=LFC_cycle
  Gain7 : Gain  Gain=K_A  SampleTime=LFC_cycle
  Gain8 : Gain  Gain=K_B  SampleTime=LFC_cycle
  Gain9 : Gain  Gain=AL_B  SampleTime=LFC_cycle
  Mux{11,13..15} (4 alike) : Mux  Inputs=2
  Mux4 : Mux  Inputs=6
  P_LOAD_A : Selector  InputPortWidth=2  IndexOptions=Index vector (dialog)  Indices=[1]  OutputSizes=1
  P_LOAD_B : Selector  InputPortWidth=2  IndexOptions=Index vector (dialog)  Indices=[2]  OutputSizes=1
  Product7 : Product  RndMeth=Zero  SampleTime=LFC_cycle
  Rate Limiter : RateLimiter  RisingSlewLimit=RA_B/60  FallingSlewLimit=-RA_B/60  SampleTimeMode=inherited
  Saturation : Saturate  UpperLimit=PMAX_B  LowerLimit=PMIN_B  SampleTime=LFC_cycle
  Scope{1,21,23,25,27} (5 alike) : Scope
  Sum17 : Sum  Inputs=|--  SampleTime=LFC_cycle
  Sum20 : Sum  Inputs=|++  SampleTime=LFC_cycle
  Sum21 : Sum  Inputs=|+-  SampleTime=LFC_cycle
  Sum5 : Sum  Inputs=|++  SampleTime=LFC_cycle
  To File4 : ToFile  Filename=AREA_B_FFC.mat  MatrixName=AREA_B_FFC  SampleTime=LFC_cycle
  Unit Delay3 : UnitDelay  SampleTime=LFC_cycle  HasFrameUpgradeWarning=on
  LFC指令値(MW) : Outport  VectorParamsAs1DForOutWhenUnconnected=off
  wires:
  P_LOAD_A/1 -> Gain7/1
  P_LOAD_B/1 -> Gain8/1
  Gain7/1 -> Sum17/1
  Gain8/1 -> Sum17/2
  Sum17/1 -> Product7/1
  Constant10/1 -> Embedded MATLAB Function4/2(XF_B)
  Embedded MATLAB Function4/1(y) -> Product7/2, Mux11/2
  Mux11/1 -> Scope21/1
  Sum21/1 -> Gain9/1
  Gain9/1 -> Sum20/1
  Sum20/1 -> Mux15/2, Unit Delay3/1, Embedded MATLAB Function5/1(u), Mux13/1, Mux4/2
  Unit Delay3/1 -> Sum21/2, Sum20/2
  Mux15/1 -> Scope23/1
  Mux13/1 -> Scope25/1
  Product7/1 -> Sum21/1, Mux15/1, Mux4/1
  Constant12/1 -> Embedded MATLAB Function5/2(XAR_B)
  Embedded MATLAB Function5/1(y) -> Mux13/2, Mux14/1, Discrete-Time Integrator/1, Gain1/1, Mux4/3
  Mux14/1 -> Scope27/1
  系統容量(MW)/1 -> P_LOAD_B/1, P_LOAD_A/1
  周波数偏差(Hz)/1 -> Embedded MATLAB Function4/1(u), Mux11/1, Mux4/5, Scope1/1
  Sum5/1 -> Mux14/2, Mux4/4, Rate Limiter/1
  Discrete-Time Integrator/1 -> Sum5/2
  Gain1/1 -> Sum5/1
  Rate Limiter/1 -> Saturation/1
  Mux4/1 -> To File4/1
  Saturation/1 -> LFC指令値(MW)/1, Mux4/6

== system AGC30Model_ex1_11/LFCモデル/他エリア TBC方式 ==
  系統容量(MW) : Inport
  周波数偏差(Hz) : Inport  Port=2
  連系線潮流偏差(Hz) : Inport  Port=3
  Constant11 : Constant  Value=XAR_B  SampleTime=LFC_cycle
  Discrete-Time Integrator : DiscreteIntegrator  gainval=KI_B  SampleTime=LFC_cycle  ICPrevOutput=DiscIntNeverNeededParam  ICPrevScaledInput=DiscIntNeverNeededParam
  Embedded MATLAB Function3 : MATLAB Function  TreatAsAtomicUnit=on
  Gain1 : Gain  Gain=KP_B  SampleTime=LFC_cycle
  Gain5 : Gain  Gain=K_B  SampleTime=LFC_cycle
  Gain6 : Gain  Gain=AL_B  SampleTime=LFC_cycle
  Mux{1,9..10,12} (4 alike) : Mux  Inputs=2
  Mux4 : Mux  Inputs=6
  P_LOAD_A3 : Selector  InputPortWidth=2  IndexOptions=Index vector (dialog)  Indices=[2]  OutputSizes=1
  Product6 : Product  RndMeth=Zero  SampleTime=LFC_cycle
  Rate Limiter : RateLimiter  RisingSlewLimit=RA_B/60  FallingSlewLimit=-RA_B/60  SampleTimeMode=inherited
  Saturation : Saturate  UpperLimit=PMAX_B  LowerLimit=PMIN_B  SampleTime=LFC_cycle
  Scope{1,17,19,24} (4 alike) : Scope
  Sum13 : Sum  Inputs=|--  SampleTime=LFC_cycle
  Sum14 : Sum  Inputs=|++  SampleTime=LFC_cycle
  Sum15 : Sum  Inputs=|+-  SampleTime=LFC_cycle
  Sum5 : Sum  Inputs=|++  SampleTime=LFC_cycle
  To File4 : ToFile  Filename=AREA_B_TBC.mat  MatrixName=AREA_B_TBC  SampleTime=LFC_cycle
  Unit Delay2 : UnitDelay  SampleTime=LFC_cycle  HasFrameUpgradeWarning=on
  自エリアAR : ToWorkspace  VariableName=ARout1  SampleTime=-1
      settings: Save2DSignal=2-D array (concatenate along first dimension)
  LFC指令値(MW) : Outport  VectorParamsAs1DForOutWhenUnconnected=off
  wires:
  Gain5/1 -> Product6/1
  Product6/1 -> Mux1/1, Sum13/1
  Sum15/1 -> Gain6/1
  Gain6/1 -> Sum14/1
  Sum14/1 -> Mux9/2, Unit Delay2/1, Embedded MATLAB Function3/1(u), Mux10/1, Mux4/2
  Unit Delay2/1 -> Sum15/2, Sum14/2
  P_LOAD_A3/1 -> Gain5/1
  Mux9/1 -> Scope17/1
  Mux10/1 -> Scope19/1
  Constant11/1 -> Embedded MATLAB Function3/2(XAR_B)
  Embedded MATLAB Function3/1(y) -> Mux10/2, Mux12/1, Discrete-Time Integrator/1, Gain1/1, Mux4/3
  Mux12/1 -> Scope24/1
  系統容量(MW)/1 -> P_LOAD_A3/1
  Discrete-Time Integrator/1 -> Sum5/2
  Gain1/1 -> Sum5/1
  Rate Limiter/1 -> Saturation/1
  Mux4/1 -> To File4/1
  Saturation/1 -> LFC指令値(MW)/1, Mux4/6
  Sum5/1 -> Mux12/2, Rate Limiter/1, Mux4/4
  連系線潮流偏差(Hz)/1 -> Mux1/2, Sum13/2
  周波数偏差(Hz)/1 -> Mux4/5, Product6/2
  Mux1/1 -> Scope1/1
  Sum13/1 -> Sum15/1, 自エリアAR/1, Mux9/1, Mux4/1

== system AGC30Model_ex1_11/LFCモデル/自エリア TBC方式 ==
  系統容量(MW) : Inport
  周波数偏差(Hz) : Inport  Port=2
  連系線潮流偏差(MW) : Inport  Port=3
  "  2" : FromFile  FileName=g_mode_input  SampleTime=dtload
  Aea A ARout : ToWorkspace  VariableName=ARout  SampleTime=-1
      settings: Save2DSignal=2-D array (concatenate along first dimension)
  Aea A LFCout : ToWorkspace  VariableName=SumLFCout  SampleTime=-1
      settings: Save2DSignal=2-D array (concatenate along first dimension)
  Constant1 : Constant  Value=RA_A  SampleTime=LFC_cycle
  Constant2 : Constant  Value=XAR_A  SampleTime=LFC_cycle
  Constant4 : Constant  Value=0.0  SampleTime=LFC_cycle
  Constant5 : Constant  Value=1.0  SampleTime=LFC_cycle
  Discrete-Time Integrator : DiscreteIntegrator  gainval=KI_A  SampleTime=LFC_cycle  ICPrevOutput=DiscIntNeverNeededParam  ICPrevScaledInput=DiscIntNeverNeededParam
  Divide : Product  Inputs=*/  SampleTime=LFC_cycle
  Embedded MATLAB Function : MATLAB Function  TreatAsAtomicUnit=on
  Gain : Gain  Gain=K_A  SampleTime=LFC_cycle
  Gain1 : Gain  Gain=KP_A  SampleTime=LFC_cycle
  Gain2 : Gain  Gain=AL_A  SampleTime=LFC_cycle
  Mux{,1..3,5} (5 alike) : Mux  Inputs=2
  Mux4 : Mux  Inputs=6
  P_LOAD_A : Selector  InputPortWidth=2  IndexOptions=Index vector (dialog)  Indices=[1]  OutputSizes=1
  Product : Product  RndMeth=Zero  SampleTime=LFC_cycle
  Product1 : Product  RndMeth=Zero  SampleTime=LFC_cycle
  Product2 : Product  RndMeth=Zero  SampleTime=LFC_cycle
  Rate Limiter : RateLimiter  RisingSlewLimit=RA_A/60  FallingSlewLimit=-RA_A/60  SampleTimeMode=inherited
  Rate Transition1 : RateTransition  OutPortSampleTime=LFC_cycle
  Scope{,1..2,6..7} (5 alike) : Scope
  Sum of Elements1 : Sum  Inputs=+  SampleTime=LFC_cycle
  Sum of Elements2 : Sum  Inputs=+  SampleTime=LFC_cycle
  Sum of Elements3 : Sum  Inputs=+  SampleTime=LFC_cycle
  Sum2 : Sum  Inputs=|-+  SampleTime=LFC_cycle
  Sum3 : Sum  Inputs=|++  SampleTime=LFC_cycle
  Sum4 : Sum  Inputs=|+-  SampleTime=LFC_cycle
  Sum5 : Sum  Inputs=|++  SampleTime=LFC_cycle
  Switch : Switch  Threshold=2  SampleTime=LFC_cycle
  To File4 : ToFile  Filename=AREA_A_TBC.mat  MatrixName=AREA_A_TBC  SampleTime=LFC_cycle
  Unit Delay : UnitDelay  SampleTime=LFC_cycle  HasFrameUpgradeWarning=on
  LFC指令値(MW) : Outport  VectorParamsAs1DForOutWhenUnconnected=off
  wires:
  Mux3/1 -> Scope7/1
  Sum of Elements2/1 -> Mux2/2
  Mux2/1 -> Scope6/1
  Product2/1 -> Sum of Elements1/1, Divide/1
  Constant5/1 -> Switch/1
  Rate Transition1/1 -> Switch/2
  Switch/1 -> Product2/2
  Constant4/1 -> Switch/3
  Product1/1 -> Sum of Elements2/1, Rate Limiter/1
  Divide/1 -> Product1/2
  Sum of Elements1/1 -> Divide/2
  Constant1/1 -> Product2/1
  Embedded MATLAB Function/1(y) -> Mux1/2, Mux4/3, Mux3/1, Discrete-Time Integrator/1, Gain1/1
  Constant2/1 -> Embedded MATLAB Function/2(XAR_A)
  Sum2/1 -> Sum4/1, Aea A ARout/1, Mux/1, Mux4/1
  Mux1/1 -> Scope2/1
  Mux/1 -> Scope/1
  P_LOAD_A/1 -> Gain/1
  Unit Delay/1 -> Sum4/2, Sum3/2
  Sum3/1 -> Mux/2, Embedded MATLAB Function/1(u), Mux1/1, Mux4/2, Unit Delay/1
  Gain2/1 -> Sum3/1
  Sum4/1 -> Gain2/1
  連系線潮流偏差(MW)/1 -> Mux5/2, Sum2/2
  Product/1 -> Mux5/1, Sum2/1
  Gain/1 -> Product/1
  系統容量(MW)/1 -> P_LOAD_A/1
  Mux4/1 -> To File4/1
  周波数偏差(Hz)/1 -> Product/2, Mux4/5
  Sum5/1 -> Mux3/2, Product1/1, Mux2/1, Mux4/4
  Discrete-Time Integrator/1 -> Sum5/2
  Gain1/1 -> Sum5/1
  "  2"/1 -> Rate Transition1/1
  Sum of Elements3/1 -> Aea A LFCout/1
  Mux5/1 -> Scope1/1
  Rate Limiter/1 -> LFC指令値(MW)/1, Mux4/6, Sum of Elements3/1

== system AGC30Model_ex1_11/LFCモデル/自エリアFFC方式 ==
  系統容量(MW) : Inport
  周波数偏差(Hz) : Inport  Port=2
  "  2" : FromFile  FileName=g_mode_input  SampleTime=dtload
  Constant1 : Constant  Value=RA_A  SampleTime=LFC_cycle
  Constant2 : Constant  Value=XAR_A  SampleTime=LFC_cycle
  Constant3 : Constant  Value=XF_A  SampleTime=LFC_cycle
  Constant4 : Constant  Value=0.0  SampleTime=LFC_cycle
  Constant5 : Constant  Value=1.0  SampleTime=LFC_cycle
  Discrete-Time Integrator : DiscreteIntegrator  gainval=KI_A  SampleTime=LFC_cycle  ICPrevOutput=DiscIntNeverNeededParam  ICPrevScaledInput=DiscIntNeverNeededParam
  Divide : Product  Inputs=*/  SampleTime=LFC_cycle
  Embedded MATLAB Function : MATLAB Function  TreatAsAtomicUnit=on
  Embedded MATLAB Function1 : MATLAB Function  TreatAsAtomicUnit=on
  Gain1 : Gain  Gain=KP_A  SampleTime=LFC_cycle
  Gain2 : Gain  Gain=AL_A  SampleTime=LFC_cycle
  Gain3 : Gain  Gain=K_A  SampleTime=LFC_cycle
  Gain4 : Gain  Gain=K_B  SampleTime=LFC_cycle
  Mux{,1..3,8} (5 alike) : Mux  Inputs=2
  Mux4 : Mux  Inputs=6
  P_LOAD_A : Selector  InputPortWidth=2  IndexOptions=Index vector (dialog)  Indices=[1]  OutputSizes=1
  P_LOAD_B : Selector  InputPortWidth=2  IndexOptions=Index vector (dialog)  Indices=[2]  OutputSizes=1
  Product1 : Product  RndMeth=Zero  SampleTime=LFC_cycle
  Product2 : Product  RndMeth=Zero  SampleTime=LFC_cycle
  Product3 : Product  RndMeth=Zero  SampleTime=LFC_cycle
  Rate Limiter : RateLimiter  RisingSlewLimit=RA_A/60  FallingSlewLimit=-RA_A/60  SampleTimeMode=inherited
  Rate Transition1 : RateTransition  OutPortSampleTime=LFC_cycle
  Scope{,2,4,6..7,16} (6 alike) : Scope
  Sum of Elements1 : Sum  Inputs=+  SampleTime=LFC_cycle
  Sum of Elements2 : Sum  Inputs=+  SampleTime=LFC_cycle
  Sum10 : Sum  Inputs=|--  SampleTime=LFC_cycle
  Sum3 : Sum  Inputs=|++  SampleTime=LFC_cycle
  Sum4 : Sum  Inputs=|+-  SampleTime=LFC_cycle
  Sum5 : Sum  Inputs=|++  SampleTime=LFC_cycle
  Switch : Switch  Threshold=2  SampleTime=LFC_cycle
  To File4 : ToFile  Filename=AREA_A_FFC.mat  MatrixName=AREA_A_FFC  SampleTime=LFC_cycle
  Unit Delay : UnitDelay  SampleTime=LFC_cycle  HasFrameUpgradeWarning=on
  LFC指令値(MW) : Outport  VectorParamsAs1DForOutWhenUnconnected=off
  wires:
  Mux3/1 -> Scope7/1
  Sum of Elements2/1 -> Mux2/2
  Mux2/1 -> Scope6/1
  Product2/1 -> Sum of Elements1/1, Divide/1
  Constant5/1 -> Switch/1
  Rate Transition1/1 -> Switch/2
  Switch/1 -> Scope4/1, Product2/2
  Constant4/1 -> Switch/3
  "  2"/1 -> Rate Transition1/1
  Product1/1 -> Sum of Elements2/1, Rate Limiter/1
  Divide/1 -> Product1/2
  Sum of Elements1/1 -> Divide/2
  Constant1/1 -> Product2/1
  Embedded MATLAB Function/1(y) -> Mux1/2, Mux4/3, Mux3/1, Discrete-Time Integrator/1, Gain1/1
  Constant2/1 -> Embedded MATLAB Function/2(XAR_A)
  Mux1/1 -> Scope2/1
  Mux/1 -> Scope/1
  Unit Delay/1 -> Sum4/2, Sum3/2
  Sum3/1 -> Mux/2, Embedded MATLAB Function/1(u), Mux1/1, Mux4/2, Unit Delay/1
  Gain2/1 -> Sum3/1
  Sum4/1 -> Gain2/1
  Mux4/1 -> To File4/1
  Rate Limiter/1 -> LFC指令値(MW)/1, Mux4/6
  Sum5/1 -> Mux3/2, Product1/1, Mux2/1, Mux4/4
  Discrete-Time Integrator/1 -> Sum5/2
  Gain1/1 -> Sum5/1
  Product3/1 -> Sum4/1, Mux/1, Mux4/1
  周波数偏差(Hz)/1 -> Embedded MATLAB Function1/1(u), Mux8/1, Mux4/5
  P_LOAD_A/1 -> Gain3/1
  P_LOAD_B/1 -> Gain4/1
  Gain3/1 -> Sum10/1
  Gain4/1 -> Sum10/2
  Sum10/1 -> Product3/1
  Constant3/1 -> Embedded MATLAB Function1/2(XF_A)
  Embedded MATLAB Function1/1(y) -> Product3/2, Mux8/2
  Mux8/1 -> Scope16/1
  系統容量(MW)/1 -> P_LOAD_A/1, P_LOAD_B/1
